simulink model "TestFlightSim1D_g_m_d"  (R2020b)
settings: Solver=VariableStepAuto  StartTime=0.0  StopTime=25  RelTol=1e-10
libraries: aerolibatmos2 x1
settings Model: Creator=jonathan  LastModifiedBy=jonathan

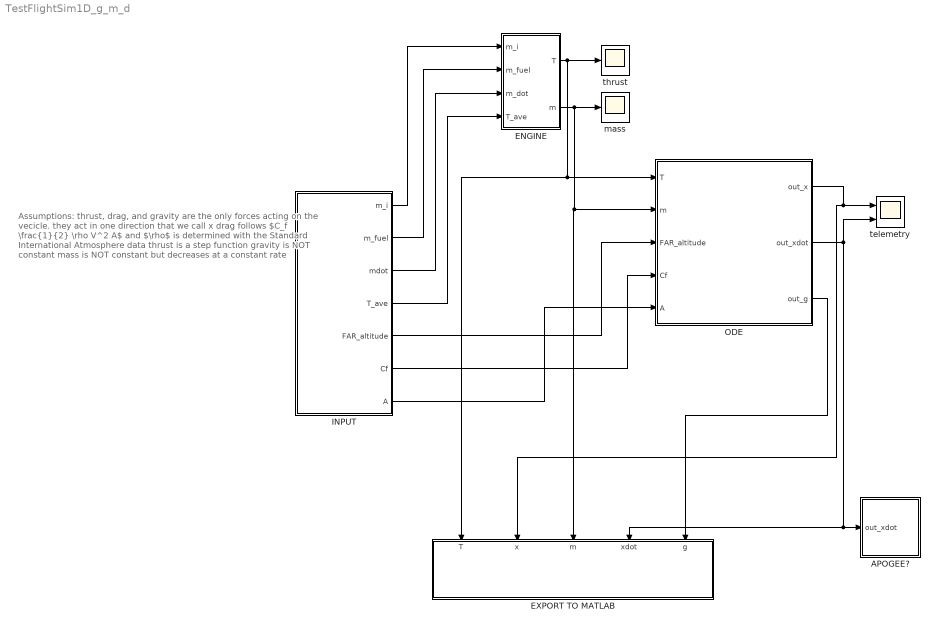
== system TestFlightSim1D_g_m_d ==
  note: Assumptions:
      | thrust, drag, and gravity are the only forces acting on the vecicle. they act in one direction that we call x
      | drag follows $C_f \frac{1}{2} \rho V^2 A$ and $\rho$ is determined with the Standard International Atmosphere data
      | thrust is a step function
      | gravity is NOT constant
      | mass is NOT constant but decreases at a constant rate
  APOGEE? : Subsystem
  ENGINE : Subsystem
  EXPORT TO MATLAB : Subsystem
  INPUT : MATLAB Function  TreatAsAtomicUnit=on
  ODE : Subsystem
  mass : Scope
  telemetry : Scope  NumInputPorts=2
  thrust : Scope
  wires:
  ODE/2(out_xdot) -> telemetry/2, APOGEE?/1(out_xdot), EXPORT TO MATLAB/4(xdot)
  ODE/1(out_x) -> telemetry/1, EXPORT TO MATLAB/2(x)
  INPUT/5(FAR_altitude) -> ODE/3(FAR_altitude)
  INPUT/4(T_ave) -> ENGINE/4(T_ave)
  INPUT/1(m_i) -> ENGINE/1(m_i)
  INPUT/2(m_fuel) -> ENGINE/2(m_fuel)
  INPUT/3(mdot) -> ENGINE/3(m_dot)
  ENGINE/1(T) -> EXPORT TO MATLAB/1(T), ODE/1(T), thrust/1
  ENGINE/2(m) -> EXPORT TO MATLAB/3(m), ODE/2(m), mass/1
  ODE/3(out_g) -> EXPORT TO MATLAB/5(g)
  INPUT/6(Cf) -> ODE/4(Cf)
  INPUT/7(A) -> ODE/5(A)

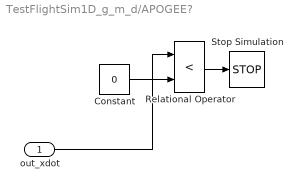
== system TestFlightSim1D_g_m_d/APOGEE? ==
  out_xdot : Inport
  Constant : Constant  Value=0
  Relational Operator : RelationalOperator  Operator=<  OutDataTypeStr=boolean  RndMeth=Simplest
  Stop Simulation : Stop
  wires:
  out_xdot/1 -> Relational Operator/1
  Constant/1 -> Relational Operator/2
  Relational Operator/1 -> Stop Simulation/1

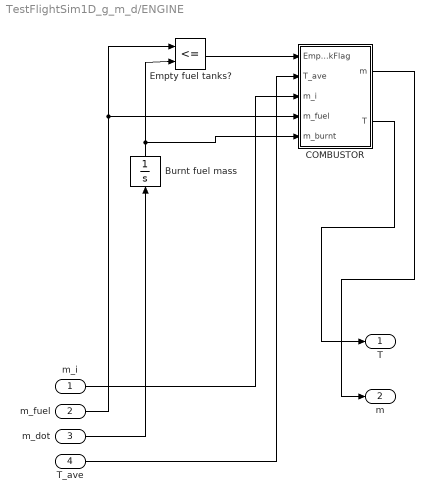
== system TestFlightSim1D_g_m_d/ENGINE ==
  m_i : Inport
  m_fuel : Inport  Port=2
  m_dot : Inport  Port=3
  T_ave : Inport  Port=4
  Burnt fuel mass : Integrator
  COMBUSTOR : MATLAB Function  TreatAsAtomicUnit=on
  Empty fuel tanks? : RelationalOperator  Operator=<=  OutDataTypeStr=boolean  RndMeth=Simplest
  T : Outport
  m : Outport  Port=2
  wires:
  COMBUSTOR/1(m) -> m/1
  T_ave/1 -> COMBUSTOR/2(T_ave)
  COMBUSTOR/2(T) -> T/1
  m_fuel/1 -> COMBUSTOR/4(m_fuel), Empty fuel tanks?/1
  m_dot/1 -> Burnt fuel mass/1
  Burnt fuel mass/1 -> Empty fuel tanks?/2, COMBUSTOR/5(m_burnt)
  m_i/1 -> COMBUSTOR/3(m_i)
  Empty fuel tanks?/1 -> COMBUSTOR/1(EmptyTankFlag)

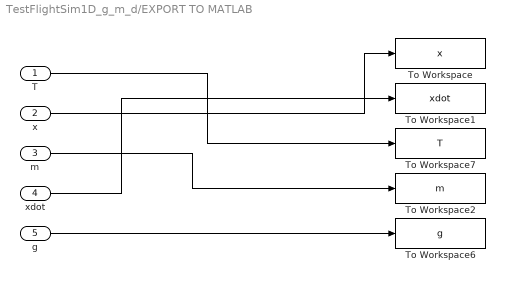
== system TestFlightSim1D_g_m_d/EXPORT TO MATLAB ==
  T : Inport
  x : Inport  Port=2
  m : Inport  Port=3
  xdot : Inport  Port=4
  g : Inport  Port=5
  To Workspace : ToWorkspace  VariableName=x  SaveFormat=Timeseries  SampleTime=-1
  To Workspace1 : ToWorkspace  VariableName=xdot  SaveFormat=Timeseries  SampleTime=-1
  To Workspace2 : ToWorkspace  VariableName=m  SaveFormat=Timeseries  SampleTime=-1
  To Workspace6 : ToWorkspace  VariableName=g  SaveFormat=Timeseries  SampleTime=-1
  To Workspace7 : ToWorkspace  VariableName=T  SaveFormat=Timeseries  SampleTime=-1
  wires:
  xdot/1 -> To Workspace1/1
  T/1 -> To Workspace7/1
  x/1 -> To Workspace/1
  m/1 -> To Workspace2/1
  g/1 -> To Workspace6/1

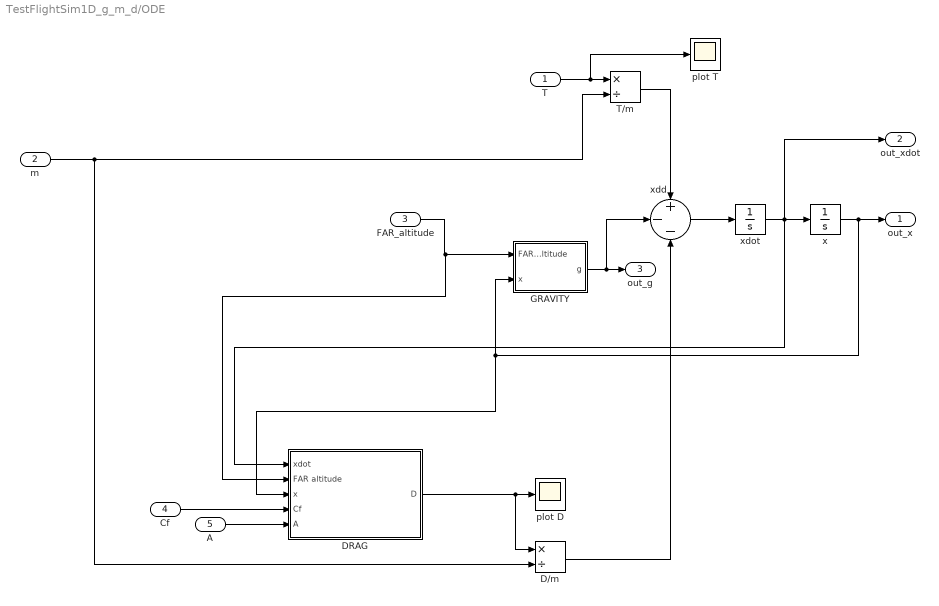
== system TestFlightSim1D_g_m_d/ODE ==
  T : Inport
  m : Inport  Port=2
  FAR_altitude : Inport  Port=3
  Cf : Inport  Port=4
  A : Inport  Port=5
  D/m : Product  Inputs=*/
  DRAG : Subsystem
  GRAVITY : MATLAB Function  TreatAsAtomicUnit=on
  T/m : Product  Inputs=*/
  "plot D " : Scope
  plot T : Scope
  x : Integrator
  xdd : Sum  Inputs=+--
  xdot : Integrator
  out_x : Outport
  out_xdot : Outport  Port=2
  out_g : Outport  Port=3
  wires:
  m/1 -> T/m/2, D/m/2
  T/1 -> plot T/1, T/m/1
  x/1 -> DRAG/3(x), GRAVITY/2(x), out_x/1
  xdot/1 -> DRAG/1(xdot), out_xdot/1, x/1
  T/m/1 -> xdd/1
  xdd/1 -> xdot/1
  FAR_altitude/1 -> DRAG/2(FAR altitude), GRAVITY/1(FAR_altitude)
  GRAVITY/1(g) -> out_g/1, xdd/2
  D/m/1 -> xdd/3
  Cf/1 -> DRAG/4(Cf)
  A/1 -> DRAG/5(A)
  DRAG/1(D) -> "plot D "/1, D/m/1

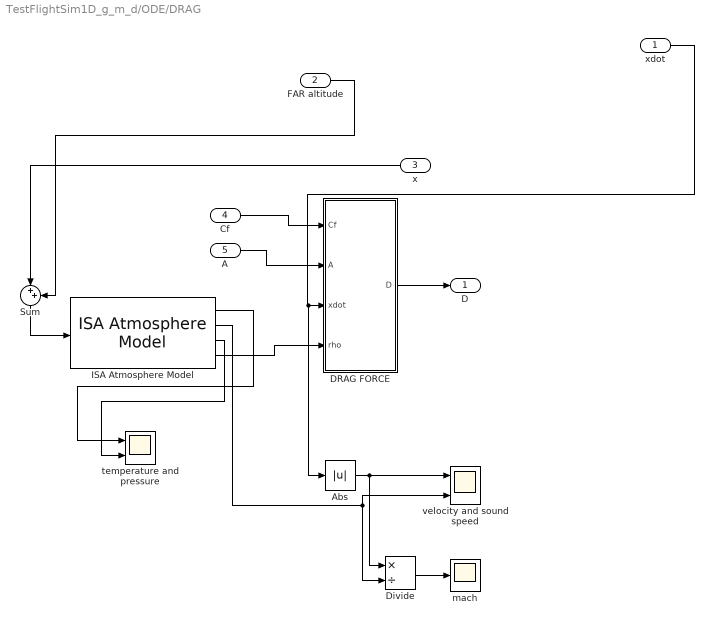
== system TestFlightSim1D_g_m_d/ODE/DRAG ==
  xdot : Inport
  FAR altitude : Inport  Port=2
  x : Inport  Port=3
  Cf : Inport  Port=4
  A : Inport  Port=5
  Abs : Abs
  DRAG FORCE : MATLAB Function  TreatAsAtomicUnit=on
  Divide : Product  Inputs=*/  RndMeth=Zero  SaturateOnIntegerOverflow=on
  ISA Atmosphere Model : aerolibatmos2/ISA Atmosphere Model  custom=off  g=9.80665  gamma=1.4  R=287.0531  L=0.0065  h_trop=11000  h_strat=20000  rho0=1.225  P0=101325  T0=288.15  h0=0
  Sum : Sum  Inputs=|++
  mach : Scope
  temperature and pressure : Scope  NumInputPorts=2
  velocity and sound speed : Scope  NumInputPorts=2
  D : Outport
  wires:
  FAR altitude/1 -> Sum/2
  DRAG FORCE/1(D) -> D/1
  ISA Atmosphere Model/4 -> DRAG FORCE/4(rho)
  Sum/1 -> ISA Atmosphere Model/1
  xdot/1 -> Abs/1, DRAG FORCE/3(xdot)
  A/1 -> DRAG FORCE/2(A)
  x/1 -> Sum/1
  Cf/1 -> DRAG FORCE/1(Cf)
  ISA Atmosphere Model/2 -> velocity and sound speed/2, Divide/2
  Abs/1 -> Divide/1, velocity and sound speed/1
  Divide/1 -> mach/1
  ISA Atmosphere Model/3 -> temperature and pressure/2
  ISA Atmosphere Model/1 -> temperature and pressure/1

== matlab function TestFlightSim1D_g_m_d/ENGINE/COMBUSTOR ==
  data: m output; EmptyTankFlag input; T output; T_ave input; m_i input; m_fuel input; m_burnt input
function [m,T] = fcn(EmptyTankFlag, T_ave, m_i, m_fuel, m_burnt)
if EmptyTankFlag == 0
    T = T_ave;
    m = m_i - m_burnt;
else
    T = 0;
    m = m_i - m_fuel;
end

end

== matlab function TestFlightSim1D_g_m_d/INPUT ==
  data: m_i output; m_fuel output; mdot output; T_ave output; FAR_altitude output; Cf output; A output
function [m_i,m_fuel,mdot,T_ave,FAR_altitude,Cf,A] = fcn
% m_i - initial vehicle mass (assumed constant)
% m_fuel - fuel mass
% mdot - mass flow rate
% T_ave - average thrust
% FAR_altitude - altitude at FAR
% Cf - coefficient of friction of rocket
% A - cross section of rocket

m_i = 200*0.453592; % [kg]
m_fuel = 34*0.453592; % [kg]
T_ave = 880*4.45; % [N]
ISP = 151; % [kg] specific impulse of rocket engine
FAR_altitude = 1068.0192; % [m] altitude of Ransburg, CA
Cf = 0.35;
A = pi*(0.161925^2); % [m2]

% calculate mass flow rate
mdot = T_ave / (ISP * 9.8); % [kg/s]

end

== matlab function TestFlightSim1D_g_m_d/ODE/GRAVITY ==
  data: FAR_altitude input; g output; x input
function g = fcn(FAR_altitude,x)

RE = 6378e3; % [m] earth sea level radius
Mu_E = 3.986e14; % [m3/s2] gravitational parameter of earth

r = RE + FAR_altitude + x;

g = Mu_E*r^(-2);

end

== matlab function TestFlightSim1D_g_m_d/ODE/DRAG/DRAG FORCE ==
  data: Cf input; A input; D output; xdot input; rho input
function D = fcn(Cf,A,xdot,rho)
% find current air density from International Standard Atmosphere 

% use drag equation
D = Cf * (1/2) * rho * (xdot^2) * A;

% make sure drag points in the right direction
if xdot < 0
    D = -D;
end

end
